simulink model "forced_msd_test"  (Simulink 7.8)
settings: Solver=ode4  StartTime=0.0  StopTime=time_span  RelTol=1e-3
undefined symbols (not defined in the file or in its folder): input_set, outstr, samp_time
libraries: simulink x1
settings Model: Creator=Kourosh Danai  LastModifiedBy=Bill
settings DataIOCC: TimeSaveName=t  OutputSaveName=y
settings DebuggingCC: AlgebraicLoopMsg=none  FcnCallInpInsideContextMsg=Use local settings  StrictBusMsg=Warning
settings SFSimCC: SimParseCustomCode=off

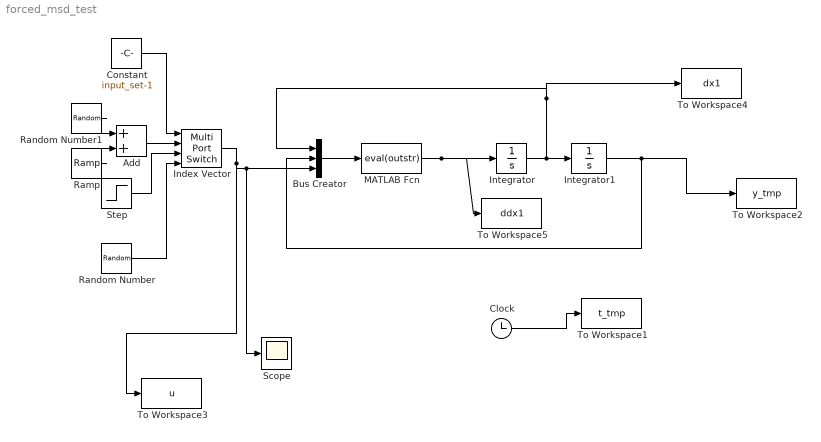
== system forced_msd_test ==
  Add : Sum
  Bus Creator : BusCreator  Inputs=3
  Clock : Clock
  Constant : Constant  Value=input_set-1  SampleTime=samp_time
  Index Vector : MultiPortSwitch  DataPortOrder=Zero-based contiguous  zeroidx=on
  Integrator : Integrator
  Integrator1 : Integrator
  MATLAB Fcn : MATLABFcn  MATLABFcn=eval(outstr)
  Ramp : simulink/Sources/Ramp  slope=10  start=0  X0=0
  Random Number : RandomNumber  Variance=1000  Seed=546  SampleTime=samp_time
  Random Number1 : RandomNumber  Variance=500  Seed=546  SampleTime=samp_time
  Scope : Scope
  Step : Step  Time=0  After=100  SampleTime=samp_time
  To Workspace1 : ToWorkspace  VariableName=t_tmp  SampleTime=samp_time  SaveFormat=Array
  To Workspace2 : ToWorkspace  VariableName=y_tmp  SampleTime=samp_time  SaveFormat=Array
  To Workspace3 : ToWorkspace  VariableName=u  SampleTime=-1  SaveFormat=Array
  To Workspace4 : ToWorkspace  VariableName=dx1  SampleTime=samp_time  SaveFormat=Array
  To Workspace5 : ToWorkspace  VariableName=ddx1  SampleTime=samp_time  SaveFormat=Array
  wires:
  Integrator/1 -> Integrator1/1, Bus Creator/1, To Workspace4/1
  Bus Creator/1 -> MATLAB Fcn/1
  Constant/1 -> Index Vector/1
  Index Vector/1 -> Bus Creator/3, Scope/1, To Workspace3/1
  Clock/1 -> To Workspace1/1
  Random Number/1 -> Index Vector/4
  Integrator1/1 -> Bus Creator/2, To Workspace2/1
  MATLAB Fcn/1 -> Integrator/1, To Workspace5/1
  Step/1 -> Index Vector/3
  Random Number1/1 -> Add/1
  Ramp/1 -> Add/2
  Add/1 -> Index Vector/2
